simulink model "Lab_4_sim_popr"  (R2021b)
settings: Solver=VariableStepAuto  StartTime=0.0  StopTime=czas_symulacji  RelTol=1e-3
values from neighbouring files (symbols this model uses):
  Cvp = cp * rop * Vp    (= 14400)    [Lab_4.m]
  Cvw = cp * rop * Vw    (= 43200)    [Lab_4.m]
  dqg = 0    [Lab_4.m]
  dTzew = 0    [Lab_4.m]
  Kcp = (qgN*a_wspol*(TwewN-TpN))/((TwewN*(1+a_wspol)-TzewN-a_wspol*TpN)*(TpN-TzewN))    (= 19.6078431373)    [Lab_4.m]
  Kcw = qgN/(TwewN*(1+a_wspol)-TzewN-a_wspol*TpN)    (= 235.294117647)    [Lab_4.m]
  Kcwp = a_wspol*Kcw    (= 58.8235294118)    [Lab_4.m]
  qg0 = qgN*0.5    (= 5000)    [Lab_4.m]
  t0 = 1000    [Lab_4.m]
  Tp0 = (Kcp*Tzew0+Kcwp*Twew0)/(Kcwp+Kcp)    (= -5)    [Lab_4.m]
  Twew0 = qg0*(Kcwp+Kcp)/(Kcw*Kcwp+Kcw*Kcp+Kcwp*Kcp) + Tzew0    (= 3.5527136788e-15)    [Lab_4.m]
  Tzew0 = TzewN    (= -20)    [Lab_4.m]
settings Model: Creator=Ovocsiak  LastModifiedBy=Ovocsiak
settings DataIOCC: ReturnWorkspaceOutputs=off

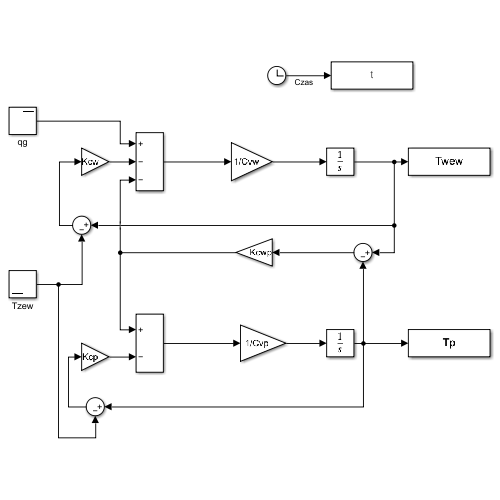
[thumbnail: Simulink's stored preview of the top-level diagram]
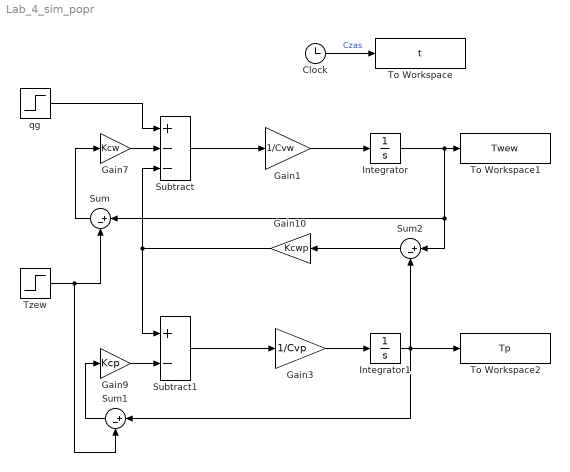
== system Lab_4_sim_popr ==
  Clock : Clock
  Gain1 : Gain  Gain=1/Cvw
  Gain10 : Gain  Gain=Kcwp
  Gain3 : Gain  Gain=1/Cvp
  Gain7 : Gain  Gain=Kcw
  Gain9 : Gain  Gain=Kcp
  Integrator : Integrator  InitialCondition=Twew0
  Integrator1 : Integrator  InitialCondition=Tp0
  Subtract : Sum  Inputs=+--
  Subtract1 : Sum  Inputs=+-
  Sum : Sum  Inputs=|+-
  Sum1 : Sum  Inputs=|+-
  Sum2 : Sum  Inputs=|+-
  To Workspace : ToWorkspace  VariableName=t  SampleTime=-1
  To Workspace1 : ToWorkspace  VariableName=Twew  SampleTime=-1
  To Workspace2 : ToWorkspace  VariableName=Tp  SampleTime=-1
  Tzew : Step  Time=t0  Before=Tzew0  After=Tzew0 + dTzew  SampleTime=0
  qg : Step  Time=t0  Before=qg0  After=qg0 + dqg  SampleTime=0
  wires:
  Clock/1 -> To Workspace/1  "Czas"
  Integrator/1 -> Sum/1, Sum2/1, To Workspace1/1
  Integrator1/1 -> Sum1/1, Sum2/2, To Workspace2/1
  qg/1 -> Subtract/1
  Subtract/1 -> Gain1/1
  Gain1/1 -> Integrator/1
  Subtract1/1 -> Gain3/1
  Gain3/1 -> Integrator1/1
  Gain7/1 -> Subtract/2
  Sum/1 -> Gain7/1
  Tzew/1 -> Sum/2, Sum1/2
  Gain10/1 -> Subtract1/1, Subtract/3
  Sum2/1 -> Gain10/1
  Gain9/1 -> Subtract1/2
  Sum1/1 -> Gain9/1
